simulink model "mtor_a"  (R2023a)
settings: Solver=FixedStepAuto  StartTime=0.0  StopTime=inf  FixedStep=0.01  RelTol=1e-3
values from neighbouring files (symbols this model uses):
  den_Gd = Gd.Den{:}    [para.m]
  encoder_scale = 1/12/4 *2*pi    (= 0.1308996939)    [para.m]
  KD = 0    [para.m]
  KI = 0.2    [para.m]
  KP = 0.05    [para.m]
  num_Gd = Gd.Num{:}    [para.m]
  Ts = 1e-2    (= 0.01)    [para.m]
  Vlim = 12    [para.m]
  Wref = 300    [para.m]
libraries: arduinolib x6, simulink x1, arduinosensorlib x1
settings Model: SimulationMode=external  ExtModeTrigDuration=2  Creator=yeoseojeong  LastModifiedBy=elec07
settings SolverCC: AutoInsertRateTranBlk=on
settings OptimizationCC: EnhancedBackFolding=on  PassReuseOutputArgsAs=Individual arguments  ZeroExternalMemoryAtStartup=off  ZeroInternalMemoryAtStartup=off  MaxStackSize=64  OptimizeBlockOrder=speed  DifferentSizesBufferReuse=on  OptimizationCustomize=off  EfficientTunableParamExpr=on
settings DebuggingCC: ParameterTunabilityLossMsg=error
settings HardwareCC: ProdBitPerInt=16  ProdBitPerPointer=16  ProdBitPerSizeT=16  ProdBitPerPtrDiffT=16  ProdLargestAtomicFloat=None  ProdWordSize=8  ProdHWDeviceType=Atmel->AVR
settings SFSimCC: MATLABDynamicMemAlloc=off
settings RTWCC: Description=Embedded Coder  SystemTargetFile=ert.tlc  HardwareBoard=Arduino Mega 2560  TemplateMakefile=ert_default_tmf  Toolchain=Arduino AVR  BuildConfiguration=Faster Runs
settings CodeAppCC: ForceParamTrailComments=on  IgnoreCustomStorageClasses=off  OperatorAnnotations=on  SimulinkDataObjDesc=on  SFDataObjDesc=on  InsertBlockDesc=on
settings ERTTargetCC: SupportContinuousTime=on  SupportVariableSizeSignals=on  ExtMode=on  ExtModeTransport=3  ExtModeStaticAlloc=on  ExtModeAutomaticAllocSize=off  ExtModeStaticAllocSize=2048  ExtModeMexFile=ext_xcp  ExtModeMexArgs=0 7 921600  ExtModeIntrfLevel=Level2 - Open

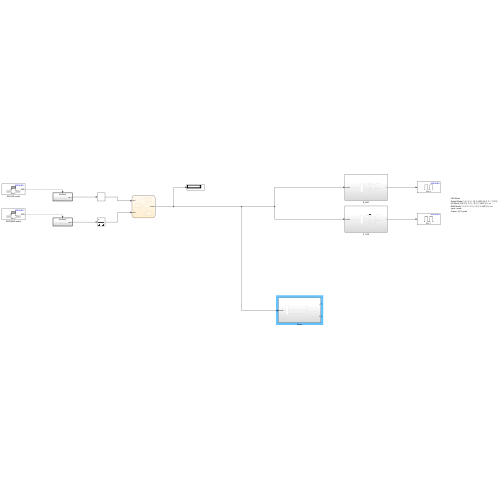
[thumbnail: Simulink's stored preview of the top-level diagram]
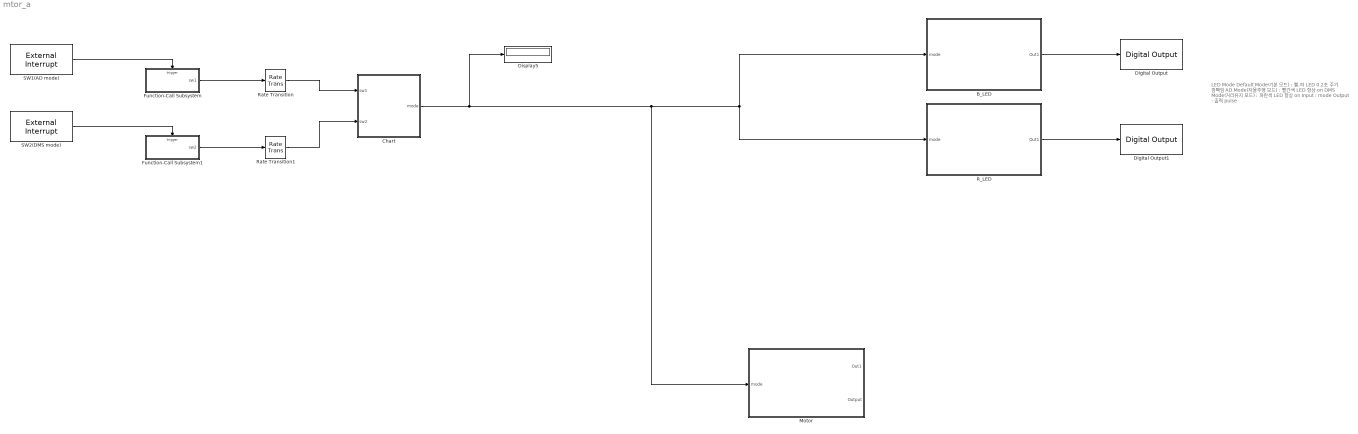
== system mtor_a ==
  note: LED Mode
      | Default Mode(기본 모드) : 빨,파 LED 0.2초 주기 깜빡임
      | AD Mode(자율주행 모드) : 빨간색 LED 항상 on
      | DMS Mode(거리유지 모드) : 파란색 LED 항상 on
      | Input : mode
      | Output : 출력 pulse
  B_LED : Subsystem
  Chart : Stateflow chart  TreatAsAtomicUnit=on
  Digital Output : arduinolib/Digital Output  pinNumber=6  Direction=output  blockPlatform=arduino
  Digital Output1 : arduinolib/Digital Output  pinNumber=7  Direction=output  blockPlatform=arduino
  Display5 : Display
  Function-Call Subsystem : Subsystem  TreatAsAtomicUnit=on
  Function-Call Subsystem1 : Subsystem  TreatAsAtomicUnit=on
  Motor : Subsystem
  R_LED : Subsystem
  Rate Transition : RateTransition  Integrity=off
  Rate Transition1 : RateTransition  Integrity=off
  SW1(AD mode) : arduinolib/External Interrupt  Pin=2  PullUp=off  Mode=RISING  InterruptSimulationInput=off
  SW2(DMS mode) : arduinolib/External Interrupt  Pin=3  PullUp=off  Mode=RISING  InterruptSimulationInput=off
  wires:
  B_LED/1(Out1) -> Digital Output/1
  R_LED/1(Out1) -> Digital Output1/1
  Function-Call Subsystem1/1(sw2) -> Rate Transition1/1
  Rate Transition/1 -> Chart/1(sw1)
  Chart/1(mode) -> Display5/1, R_LED/1(mode), B_LED/1(mode), Motor/1(mode)
  SW2(DMS mode)/1 -> Function-Call Subsystem1/Trigger
  SW1(AD mode)/1 -> Function-Call Subsystem/Trigger
  Function-Call Subsystem/1(sw1) -> Rate Transition/1
  Rate Transition1/1 -> Chart/2(sw2)

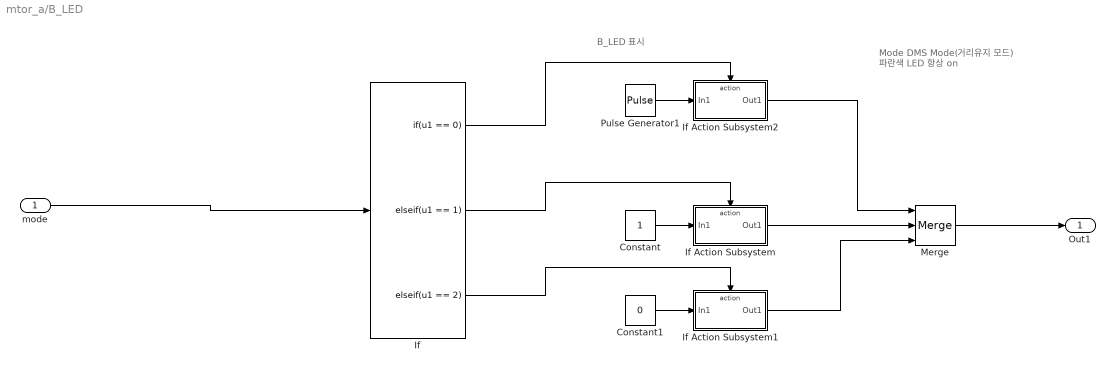
== system mtor_a/B_LED ==
  note: B_LED 표시
  note: Mode
      | DMS Mode(거리유지 모드)
      | 파란색 LED 항상 on
  mode : Inport
  Constant : Constant
  Constant1 : Constant  Value=0
  If : If  IfExpression=u1 == 0  ElseIfExpressions=u1 == 1, u1 == 2  ShowElse=off
  If Action Subsystem : Subsystem  TreatAsAtomicUnit=on
  If Action Subsystem1 : Subsystem  TreatAsAtomicUnit=on
  If Action Subsystem2 : Subsystem  TreatAsAtomicUnit=on
  Merge : Merge  Inputs=3
  Pulse Generator1 : DiscretePulseGenerator  PulseType=Time based  Period=0.4  PulseWidth=50
  Out1 : Outport
  wires:
  mode/1 -> If/1
  Constant/1 -> If Action Subsystem/1(In1)
  If Action Subsystem/1(Out1) -> Merge/2
  Merge/1 -> Out1/1
  If/2 -> If Action Subsystem/Action
  If/1 -> If Action Subsystem2/Action
  Pulse Generator1/1 -> If Action Subsystem2/1(In1)
  If Action Subsystem2/1(Out1) -> Merge/1
  Constant1/1 -> If Action Subsystem1/1(In1)
  If/3 -> If Action Subsystem1/Action
  If Action Subsystem1/1(Out1) -> Merge/3

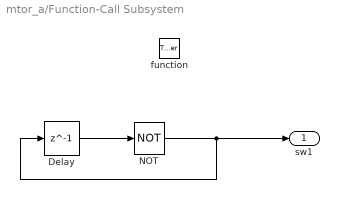
== system mtor_a/Function-Call Subsystem ==
  function : TriggerPort  TriggerType=function-call  VariantControl=(inherit)
  Delay : Delay  DelayLength=1  InitialCondition=0
  NOT : Logic  Operator=NOT  IconShape=distinctive  AllPortsSameDT=off  OutDataTypeStr=boolean
  sw1 : Outport
  wires:
  Delay/1 -> NOT/1
  NOT/1 -> Delay/1, sw1/1

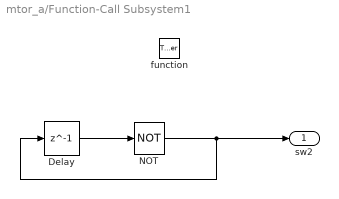
== system mtor_a/Function-Call Subsystem1 ==
  function : TriggerPort  TriggerType=function-call  VariantControl=(inherit)
  Delay : Delay  DelayLength=1  InitialCondition=0
  NOT : Logic  Operator=NOT  IconShape=distinctive  AllPortsSameDT=off  OutDataTypeStr=boolean
  sw2 : Outport
  wires:
  Delay/1 -> NOT/1
  NOT/1 -> Delay/1, sw2/1

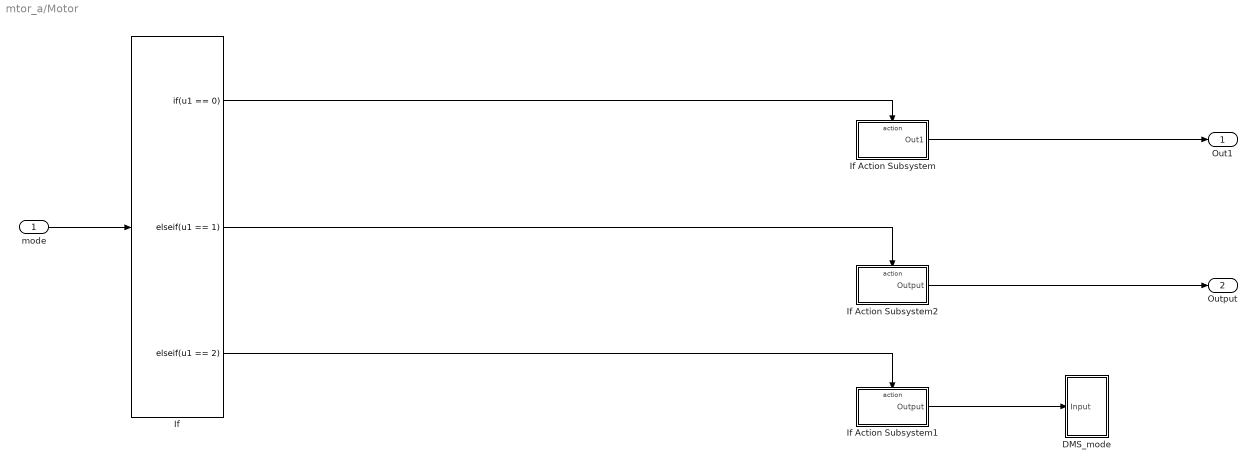
== system mtor_a/Motor ==
  mode : Inport
  DMS_mode : Subsystem
  If : If  IfExpression=u1 == 0  ElseIfExpressions=u1 == 1, u1 == 2  ShowElse=off
  If Action Subsystem : Subsystem  TreatAsAtomicUnit=on
  If Action Subsystem1 : Subsystem  TreatAsAtomicUnit=on
  If Action Subsystem2 : Subsystem  TreatAsAtomicUnit=on
  Out1 : Outport
  Output : Outport  Port=2
  wires:
  mode/1 -> If/1
  If/1 -> If Action Subsystem/Action
  If Action Subsystem/1(Out1) -> Out1/1
  If/2 -> If Action Subsystem2/Action
  If Action Subsystem2/1(Output) -> Output/1
  If/3 -> If Action Subsystem1/Action
  If Action Subsystem1/1(Output) -> DMS_mode/1(Input)

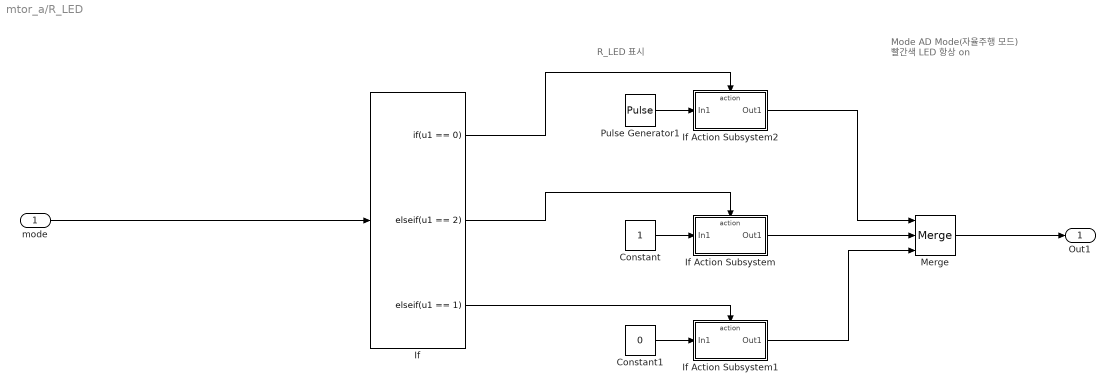
== system mtor_a/R_LED ==
  note: R_LED 표시
  note: Mode
      | AD Mode(자율주행 모드)
      | 빨간색 LED 항상 on
  mode : Inport
  Constant : Constant
  Constant1 : Constant  Value=0
  If : If  IfExpression=u1 == 0  ElseIfExpressions=u1 == 2, u1 == 1  ShowElse=off
  If Action Subsystem : Subsystem  TreatAsAtomicUnit=on
  If Action Subsystem1 : Subsystem  TreatAsAtomicUnit=on
  If Action Subsystem2 : Subsystem  TreatAsAtomicUnit=on
  Merge : Merge  Inputs=3
  Pulse Generator1 : DiscretePulseGenerator  PulseType=Time based  Period=0.4  PulseWidth=50
  Out1 : Outport
  wires:
  mode/1 -> If/1
  Constant/1 -> If Action Subsystem/1(In1)
  If Action Subsystem/1(Out1) -> Merge/2
  Merge/1 -> Out1/1
  If/2 -> If Action Subsystem/Action
  If/1 -> If Action Subsystem2/Action
  Pulse Generator1/1 -> If Action Subsystem2/1(In1)
  If Action Subsystem2/1(Out1) -> Merge/1
  If/3 -> If Action Subsystem1/Action
  Constant1/1 -> If Action Subsystem1/1(In1)
  If Action Subsystem1/1(Out1) -> Merge/3

== system mtor_a/B_LED/If Action Subsystem ==
  In1 : Inport
  Action Port : ActionPort  ActionPortLabel=elseif(u1 == 1)
  Out1 : Outport
  wires:
  In1/1 -> Out1/1

== system mtor_a/B_LED/If Action Subsystem1 ==
  In1 : Inport
  Action Port : ActionPort  ActionPortLabel=elseif( u1 == 2)
  Out1 : Outport
  wires:
  In1/1 -> Out1/1

== system mtor_a/B_LED/If Action Subsystem2 ==
  In1 : Inport
  Action Port : ActionPort  ActionPortLabel=if(u1 == 0)
  Out1 : Outport
  wires:
  In1/1 -> Out1/1

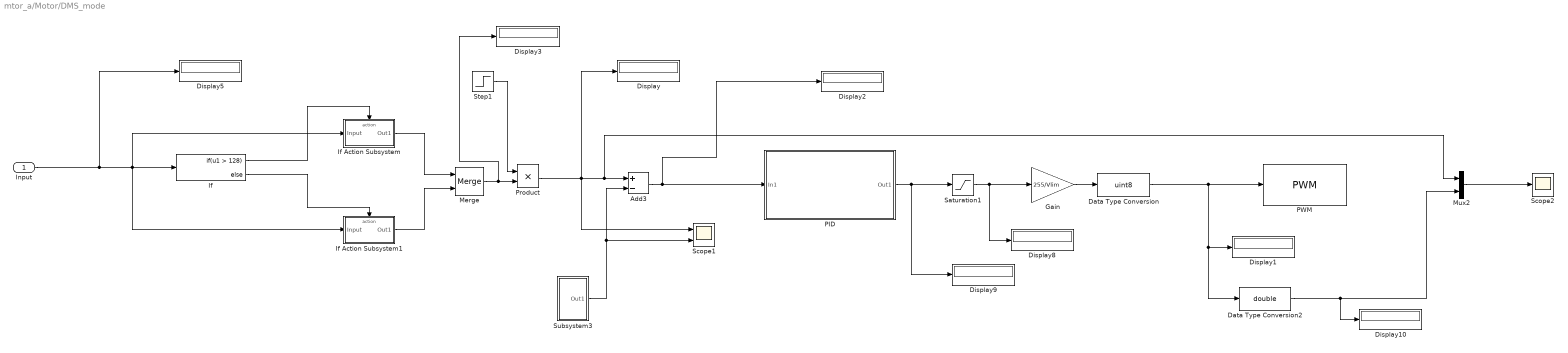
== system mtor_a/Motor/DMS_mode ==
  Input : Inport
  Add3 : Sum  Inputs=+-
  Data Type Conversion : DataTypeConversion  OutDataTypeStr=uint8  SaturateOnIntegerOverflow=off  RndMeth=Floor
  Data Type Conversion2 : DataTypeConversion  OutDataTypeStr=double  SaturateOnIntegerOverflow=off  RndMeth=Floor
  Display{,1..3,5,8..10} (8 alike) : Display
  Gain : Gain  Gain=255/Vlim
  If : If  IfExpression=u1 > 128
  If Action Subsystem : Subsystem  TreatAsAtomicUnit=on
  If Action Subsystem1 : Subsystem  TreatAsAtomicUnit=on
  Merge : Merge
  Mux2 : Mux  Inputs=2
  PID : Subsystem
  PWM : arduinolib/PWM  pinNumber=11  frequencyType=Default  desiredFrequency=490.2  achievableFrequency=490.2
  Product : Product
  Saturation1 : Saturate  UpperLimit=12  LowerLimit=0
  Scope1 : Scope  NumInputPorts=2
  Scope2 : Scope
  Step1 : Step  After=Wref  SampleTime=0
  Subsystem3 : Subsystem
  wires:
  Input/1 -> Display5/1, If Action Subsystem1/1(Input), If/1, If Action Subsystem/1(Input)
  Product/1 -> Scope1/1, Mux2/1, Add3/1, Display/1
  Step1/1 -> Product/1
  Saturation1/1 -> Gain/1, Display8/1
  Data Type Conversion2/1 -> Mux2/2, Display10/1
  PID/1(Out1) -> Display9/1, Saturation1/1
  Data Type Conversion/1 -> Display1/1, Data Type Conversion2/1, PWM/1
  Subsystem3/1(Out1) -> Scope1/2, Add3/2
  Mux2/1 -> Scope2/1
  Add3/1 -> Display2/1, PID/1(In1)
  Gain/1 -> Data Type Conversion/1
  If/1 -> If Action Subsystem/Action
  If/2 -> If Action Subsystem1/Action
  Merge/1 -> Display3/1, Product/2
  If Action Subsystem/1(Out1) -> Merge/1
  If Action Subsystem1/1(Out1) -> Merge/2

== system mtor_a/Motor/If Action Subsystem ==
  Action Port : ActionPort  ActionPortLabel=if(u1 == 0)
  Out1 : Outport

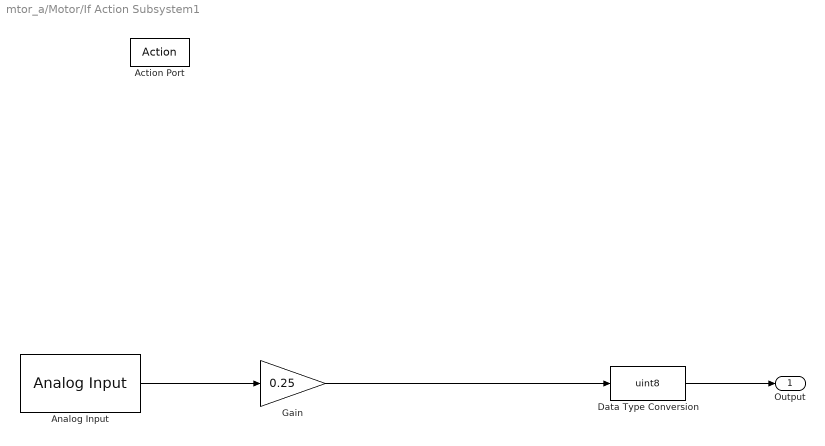
== system mtor_a/Motor/If Action Subsystem1 ==
  Action Port : ActionPort  ActionPortLabel=elseif( u1 == 2)
  Analog Input : arduinolib/Analog Input  pinNumber=2  ReadResultsOnly=off  ConversionTriggerSource=Software  ExternalTriggerType=uint32( 0 )  OutputDataType=uint16  EnableConversionCompleteNotify=off  EnableOuputStatus=off  SampleTime=-1  blockPlatform=arduino
  Data Type Conversion : DataTypeConversion  OutDataTypeStr=uint8  SaturateOnIntegerOverflow=off  RndMeth=Floor
  Gain : Gain  Gain=0.25
  Output : Outport
  wires:
  Gain/1 -> Data Type Conversion/1
  Analog Input/1 -> Gain/1
  Data Type Conversion/1 -> Output/1

== system mtor_a/Motor/If Action Subsystem2 ==
  Action Port : ActionPort  ActionPortLabel=elseif(u1 == 1)
  Output : Outport

== system mtor_a/R_LED/If Action Subsystem ==
  In1 : Inport
  Action Port : ActionPort  ActionPortLabel=elseif(u1 == 2)
  Out1 : Outport
  wires:
  In1/1 -> Out1/1

== system mtor_a/R_LED/If Action Subsystem1 ==
  In1 : Inport
  Action Port : ActionPort  ActionPortLabel=elseif( u1 == 1)
  Out1 : Outport
  wires:
  In1/1 -> Out1/1

== system mtor_a/R_LED/If Action Subsystem2 ==
  In1 : Inport
  Action Port : ActionPort  ActionPortLabel=if(u1 == 0)
  Out1 : Outport
  wires:
  In1/1 -> Out1/1

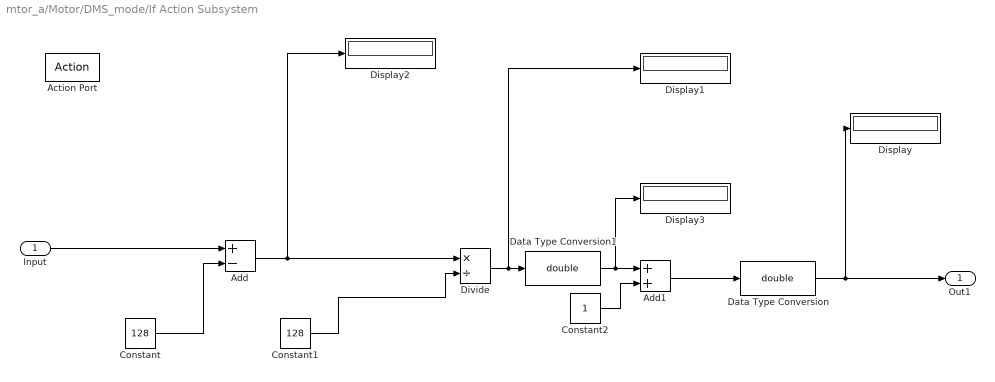
== system mtor_a/Motor/DMS_mode/If Action Subsystem ==
  Input : Inport
  Action Port : ActionPort  ActionPortLabel=if(u1 > 128)
  Add : Sum  Inputs=+-
  Add1 : Sum
  Constant : Constant  Value=128
  Constant1 : Constant  Value=128
  Constant2 : Constant
  Data Type Conversion : DataTypeConversion  OutDataTypeStr=double  SaturateOnIntegerOverflow=off  RndMeth=Floor
  Data Type Conversion1 : DataTypeConversion  OutDataTypeStr=double  SaturateOnIntegerOverflow=off  RndMeth=Floor
  Display{,1..3} (4 alike) : Display
  Divide : Product  Inputs=*/
  Out1 : Outport
  wires:
  Constant1/1 -> Divide/2
  Input/1 -> Add/1
  Constant/1 -> Add/2
  Constant2/1 -> Add1/2
  Add1/1 -> Data Type Conversion/1
  Data Type Conversion/1 -> Display/1, Out1/1
  Add/1 -> Divide/1, Display2/1
  Divide/1 -> Display1/1, Data Type Conversion1/1
  Data Type Conversion1/1 -> Display3/1, Add1/1

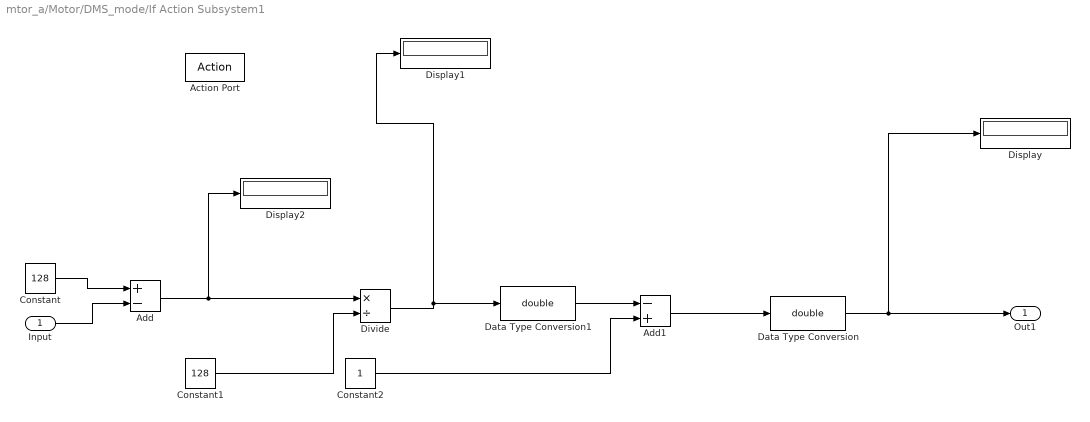
== system mtor_a/Motor/DMS_mode/If Action Subsystem1 ==
  Input : Inport
  Action Port : ActionPort  ActionPortLabel=else
  Add : Sum  Inputs=+-
  Add1 : Sum  Inputs=-+
  Constant : Constant  Value=128
  Constant1 : Constant  Value=128
  Constant2 : Constant
  Data Type Conversion : DataTypeConversion  OutDataTypeStr=double  SaturateOnIntegerOverflow=off  RndMeth=Floor
  Data Type Conversion1 : DataTypeConversion  OutDataTypeStr=double  SaturateOnIntegerOverflow=off  RndMeth=Floor
  Display : Display
  Display1 : Display
  Display2 : Display
  Divide : Product  Inputs=*/
  Out1 : Outport
  wires:
  Constant2/1 -> Add1/2
  Constant1/1 -> Divide/2
  Add1/1 -> Data Type Conversion/1
  Data Type Conversion/1 -> Display/1, Out1/1
  Constant/1 -> Add/1
  Input/1 -> Add/2
  Divide/1 -> Data Type Conversion1/1, Display1/1
  Add/1 -> Divide/1, Display2/1
  Data Type Conversion1/1 -> Add1/1

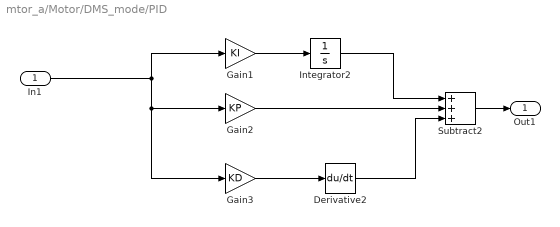
== system mtor_a/Motor/DMS_mode/PID ==
  In1 : Inport
  Derivative2 : Derivative
  Gain1 : Gain  Gain=KI
  Gain2 : Gain  Gain=KP
  Gain3 : Gain  Gain=KD
  Integrator2 : Integrator
  Subtract2 : Sum  Inputs=+++
  Out1 : Outport
  wires:
  Gain1/1 -> Integrator2/1
  Gain2/1 -> Subtract2/2
  Integrator2/1 -> Subtract2/1
  In1/1 -> Gain2/1, Gain3/1, Gain1/1
  Derivative2/1 -> Subtract2/3
  Gain3/1 -> Derivative2/1
  Subtract2/1 -> Out1/1

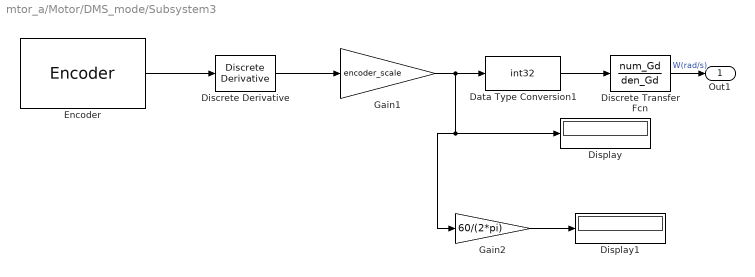
== system mtor_a/Motor/DMS_mode/Subsystem3 ==
  Data Type Conversion1 : DataTypeConversion  OutDataTypeStr=int32  SaturateOnIntegerOverflow=off  RndMeth=Floor
  Discrete Transfer Fcn : DiscreteTransferFcn  Numerator=num_Gd  Denominator=den_Gd  SampleTime=Ts
  Discrete Derivative : simulink/Discrete/Discrete Derivative  gainval=1.0  ICPrevScaledInput=0.0  InputProcessing=Columns as channels (frame based)  OutMin=[]  OutMax=[]  OutDataType=fixdt(1, 16)  OutScaling=2^-10  DoSatur=off
  Display : Display
  Display1 : Display
  Encoder : arduinosensorlib/Encoder  InputA=18  InputB=19  Mode=No reset  SampleTime=-1
  Gain1 : Gain  Gain=encoder_scale
  Gain2 : Gain  Gain=60/(2*pi)
  Out1 : Outport
  wires:
  Gain1/1 -> Gain2/1, Display/1, Data Type Conversion1/1
  Encoder/1 -> Discrete Derivative/1
  Gain2/1 -> Display1/1
  Discrete Derivative/1 -> Gain1/1
  Discrete Transfer Fcn/1 -> Out1/1  "W(rad/s)"
  Data Type Conversion1/1 -> Discrete Transfer Fcn/1

== stateflow chart mtor_a/Chart ==
  state AD_mode
    en:
    flag1 = sw1, flag2 = sw2;
    du:
    mode = 1;
  state mode_off
    en:
    flag1 = sw1, flag2 = sw2;
    du:
    mode = 0;
  state DMS_mode
    en:
    flag1 = sw1, flag2 = sw2;
    du:
    mode = 2;
  mode_off -> AD_mode [order 1] : [flag1 ~= sw1]
  AD_mode -> mode_off : [flag1 ~= sw1 || flag2 ~= sw2]
  (default) -> mode_off
  DMS_mode -> mode_off : [flag2 ~=  sw2 || flag1 ~= sw1]
  mode_off -> DMS_mode [order 2] : [flag2 ~= sw2]
  data: sw1 input; sw2 input; mode output; flag1 local; flag2 local
